simulink model "DCshuntChar"  (R2017a)
settings: Solver=VariableStepAuto  StartTime=0.0  StopTime=10.0  MaxStep=1e-4  RelTol=1e-3
libraries: simulink x4, powerlib x3, powerlib_meascontrol x2
settings Model: Creator=Matlab  LastModifiedBy=Matlab

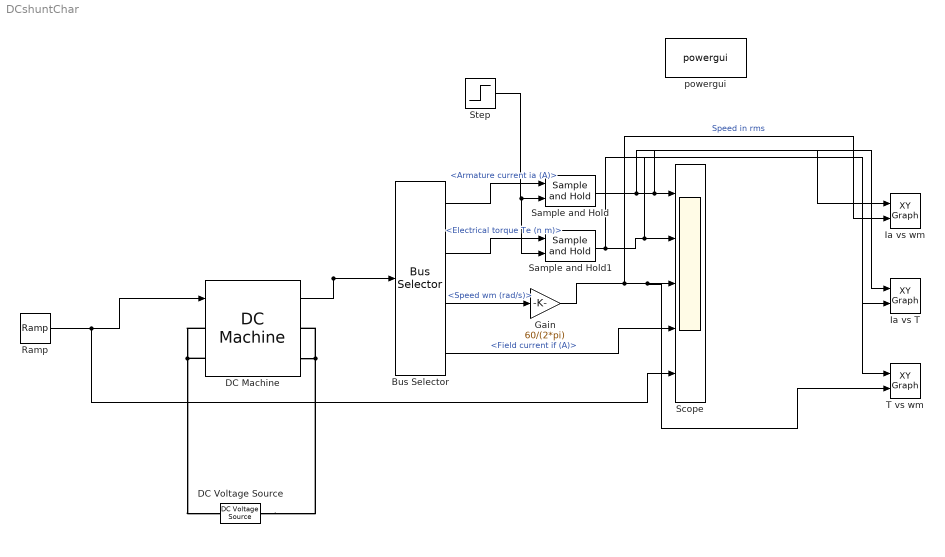
== system DCshuntChar ==
  Bus Selector : BusSelector  OutputSignals=Armature current ia (A),Electrical torque Te (n m),Speed wm (rad/s),Field current if (A)
  DC Machine : powerlib/Machines/DC Machine  PresetModel=01: 5HP 240V 1750RPM Field:300V  MechanicalLoad=Torque TL  FieldType=Wound  ShowDetailedParameters=on  MeasurementBus=off  RLa=[2.581 0.028]  RLf=[281.3 156]  Laf=0.9483  MachineConstant=Torque constant (N.m/A)  Ke=1.8  Kt=1.8  J=0.02215  Bm=0.002953  Tf=0.5161  w0=1  Ifinit=1  TsPowergui=0  TsBlock=-1
  DC Voltage Source : powerlib/Electrical Sources/DC Voltage Source  Amplitude=240  Measurements=None
  Gain : Gain  Gain=60/(2*pi)
  Ia vs T : simulink/Sinks/XY Graph  xmin=5  xmax=30  ymin=0  ymax=22  st=1
  Ia vs wm : simulink/Sinks/XY Graph  xmin=5  xmax=30  ymin=0  ymax=3000  st=1
  Ramp : simulink/Sources/Ramp  slope=2  start=0  X0=0
  Sample and Hold : powerlib_meascontrol/Additional Components/Sample and Hold  ic=0  Ts=0
      settings: SourceProductName=Simscape Power Systems  SourceProductBaseCode=PS
  Sample and Hold1 : powerlib_meascontrol/Additional Components/Sample and Hold  ic=0  Ts=0
      settings: SourceProductName=Simscape Power Systems  SourceProductBaseCode=PS
  Scope : Scope  NumInputPorts=5
  Step : Step  Time=0.5  SampleTime=0
  T vs wm : simulink/Sinks/XY Graph  xmin=5  xmax=22  ymin=0  ymax=3000  st=1
  powergui : powerlib/powergui  Priority=1  SimulationMode=Continuous  SampleTime=50e-6  frequency=60  Iterations=50  frequencyindice=0  Pbase=100e6  ErrMax=1e-4  UnitsV=kV  UnitsW=MW  buscounter=0  FunctionMessages=off  echomessages=off  EnableUseOfTLC=off  CurrentSourceSwitches=off  DisableSnubberDevices=off  DisableRonSwitches=off  DisableVfSwitches=off  DisplayEquations=off  SolverType=Tustin/Backward Euler (TBE)  Interpol=off  ExternalGateDelay=off  methode=off  Ts=100  x0status=blocks  SPID=on  SwTol=0  HookPort=off  RestoreLinks=warning  ResistiveCurrentMeasurement=off  Frange=[0:2:500]  Ylog=off  Xlog=on  ShowGrid=off  save=off  variable=ZData  structure=0  ZoomFFT=off  StartTime=0.0  cycles=1  DisplayStyle=1  fundamental=60  FreqAxis=off  MaxFrequency=1000  frequencyindicesteady=1  RmsSteady=1  display=off
  wires:
  Ramp/1 -> Scope/5, DC Machine/1
  DC Machine/1 -> Bus Selector/1
  Bus Selector/3 -> Gain/1  "<Speed wm (rad/s)>"
  Bus Selector/4 -> Scope/4  "<Field current if (A)>"
  Bus Selector/1 -> Sample and Hold/1  "<Armature current ia (A)>"
  Sample and Hold/1 -> Ia vs wm/1, Ia vs T/1, Scope/1
  Bus Selector/2 -> Sample and Hold1/1  "<Electrical torque Te (n m)>"
  Sample and Hold1/1 -> Ia vs T/2, T vs wm/1, Scope/2
  Step/1 -> Sample and Hold1/2, Sample and Hold/2
  Gain/1 -> Ia vs wm/2, T vs wm/2, Scope/3  "Speed in rms"
  connections:
  DC Machine/LConn1 -- DC Machine/LConn2 -- DC Voltage Source/RConn1
  DC Voltage Source/LConn1 -- DC Machine/RConn2 -- DC Machine/RConn1
